simulink model "HW_7_1part"  (R2022b)
settings: Solver=VariableStepAuto  StartTime=0.0  StopTime=5  RelTol=1e-3
values from neighbouring files (symbols this model uses):
  Gain = prod([dp1, dp2, dp3])/prod([dz1, dz2])/0.001708    [HW7_1part.m]
  k = 44.567    [HW7_1part.m]
  l_p = L_p(1)    [HW7_1part.m]
  l_z = L_z    [HW7_1part.m]
  mass = 0.01    [HW7_1part.m]
  Ts = 0.1    [HW7_1part.m]
settings Model: Creator=ROG  LastModifiedBy=ROG
settings DataIOCC: SaveFormat=Array

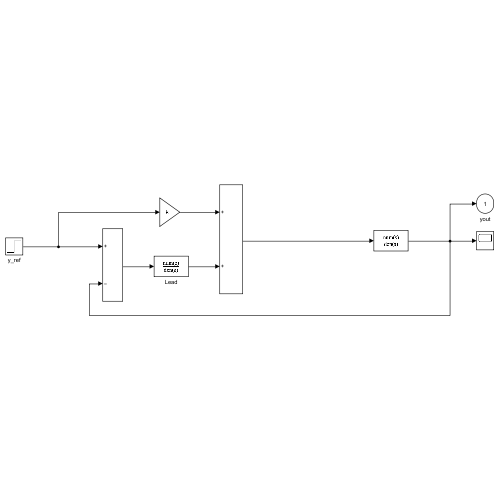
[thumbnail: Simulink's stored preview of the top-level diagram]
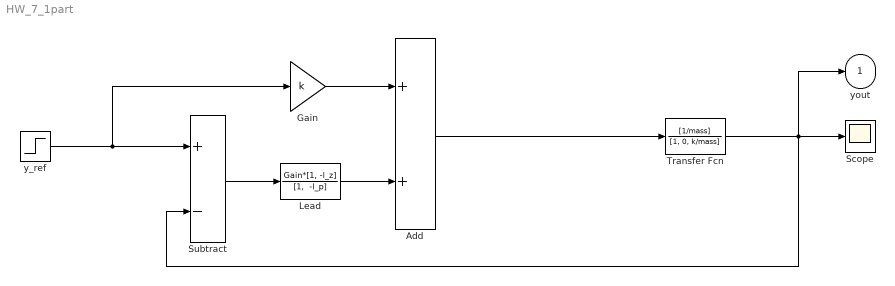
== system HW_7_1part ==
  Add : Sum
  Gain : Gain  Gain=k
  Lead : DiscreteTransferFcn  Numerator=Gain*[1, -l_z]  Denominator="[1,  -l_p]"  SampleTime=Ts
  Scope : Scope
  Subtract : Sum  Inputs=+-
  Transfer Fcn : TransferFcn  Numerator=[1/mass]  Denominator=[1, 0, k/mass]
  y_ref : Step  Time=0  SampleTime=0
  yout : Outport
  wires:
  Subtract/1 -> Lead/1
  Lead/1 -> Add/2
  Gain/1 -> Add/1
  Transfer Fcn/1 -> yout/1, Subtract/2, Scope/1
  y_ref/1 -> Gain/1, Subtract/1
  Add/1 -> Transfer Fcn/1
